simulink model "SAD_projectSamu"  (R2023b)
settings: Solver=ode4  StartTime=t0  StopTime=1000  FixedStep=t_step  RelTol=1e-3
model workspace (MAT data in the model file):
  N_order = 1
values from neighbouring files (symbols this model uses):
  A1 = importdata("igrfSg.txt")    [SAD_project_code.m]
  A2 = importdata("igrfSh.txt")    [SAD_project_code.m]
  A_1 = area_face(1)    [SAD_project_code.m]
  A_2 = area_face(2)    [SAD_project_code.m]
  A_3 = area_face(3)    [SAD_project_code.m]
  A_4 = area_face(4)    [SAD_project_code.m]
  A_5 = area_face(5)    [SAD_project_code.m]
  A_6 = area_face(6)    [SAD_project_code.m]
  alpha = [1/6 5/6]    [SAD_project_code.m]
  ARW = ARW*[1 1 1]'    [SAD_project_code.m]
  bias = bias*[1 1 1]'    [SAD_project_code.m]
  DCM_eci_per = rotationMatrix(rad2deg(i),rad2deg(OM), rad2deg(om))    [SAD_project_code.m]
  e = 0.0011241    [SAD_project_code.m]
  FS = 50000e-9    (= 5e-05)    [SAD_project_code.m]
  H0 = [g_10 g_11 h_11]'    [SAD_project_code.m]
  h_r_0 = [0,0,0]'    [SAD_project_code.m]
  horizon_cone_limit = deg2rad(350)    [SAD_project_code.m]
  I = 5/12.*diag([Ix Iy Iz])    [SAD_project_code.m]
  i = deg2rad(97.55)    [SAD_project_code.m]
  I_inv = inv(I)    [SAD_project_code.m]
  I_RW = 1e-2    (= 0.01)    [SAD_project_code.m]
  I_vector_RW = [I_RW I_RW I_RW]'    [SAD_project_code.m]
  inc_tot = sqrt(inc_lin^2 + inc_acc^2)    [SAD_project_code.m]
  InitialTrueAnomalyOfEarth = 0    [SAD_project_code.m]
  j_b = [0.001 0.005 0.001]'    [SAD_project_code.m]
  K1_point = lqr(A, B, Q, R)    [SAD_project_code.m]
  K1_slew = lqr(A,B, Q, R)    [SAD_project_code.m]
  K2_point = K1_point.^2/2    [SAD_project_code.m]
  K2_slew = K1_slew.^2/2    [SAD_project_code.m]
  K_detumbling = lqr(A,B,Q,R)    [SAD_project_code.m]
  matrix_RW_config = eye(3)    [SAD_project_code.m]
  matrix_RW_config_inv = inv(matrix_RW_config)    [SAD_project_code.m]
  mu_E = astroConstants(13)    [SAD_project_code.m]
  N_1 = BODY(1,:)    [SAD_project_code.m]
  N_2 = BODY(2,:)    [SAD_project_code.m]
  N_3 = BODY(3,:)    [SAD_project_code.m]
  N_4 = BODY(4,:)    [SAD_project_code.m]
  N_5 = BODY(5,:)    [SAD_project_code.m]
  N_6 = BODY(6,:)    [SAD_project_code.m]
  n_e = sqrt(mu_E/a^3)    [SAD_project_code.m]
  om = deg2rad(206.3209)    [SAD_project_code.m]
  OM = deg2rad(50.7464)    [SAD_project_code.m]
  p = a*(1-e^2)    [SAD_project_code.m]
  q0 = [0.1, -0.7, 0.51, 0.41]    [SAD_project_code.m]
  r_1 = r(1,:)    [SAD_project_code.m]
  r_2 = r(2,:)    [SAD_project_code.m]
  r_3 = r(3,:)    [SAD_project_code.m]
  r_4 = r(4,:)    [SAD_project_code.m]
  r_5 = r(5,:)    [SAD_project_code.m]
  r_6 = r(6,:)    [SAD_project_code.m]
  R_E = astroConstants(23)    [SAD_project_code.m]
  rho_d1 = 0.1    [SAD_project_code.m]
  rho_d2 = 0.1    [SAD_project_code.m]
  rho_d3 = 0.1    [SAD_project_code.m]
  rho_d4 = 0.1    [SAD_project_code.m]
  rho_d5 = 0.1    [SAD_project_code.m]
  rho_d6 = 0.1    [SAD_project_code.m]
  rho_s1 = rho_s(1)    [SAD_project_code.m]
  rho_s2 = rho_s(2)    [SAD_project_code.m]
  rho_s3 = rho_s(3)    [SAD_project_code.m]
  rho_s4 = rho_s(4)    [SAD_project_code.m]
  rho_s5 = rho_s(5)    [SAD_project_code.m]
  rho_s6 = rho_s(6)    [SAD_project_code.m]
  t_step = 0.01    [SAD_project_code.m]
  th0 = deg2rad(0)    [SAD_project_code.m]
  timeoflaunch = date2mjd2000(date0)    [SAD_project_code.m]
  torque_max = 0.8    [SAD_project_code.m]
  ts_sensor = 5*t_step    (= 0.05)    [SAD_project_code.m]
  w0 = [wx0 wy0 wz0]'    [SAD_project_code.m]
  w0_RW = [0 0 0]    [SAD_project_code.m]
  w_E = deg2rad(15.04)/60/60    [SAD_project_code.m]
  wMax_RW = 2*pi * RPM_max_RW / 60    (= 527.263967027)    [SAD_project_code.m]
libraries: matrix_library x43, dspindex x6, simulink x5, simulink_extras x4, sharedtransform x4, aerolibutil x2, vrlib x2, dspinverses x1
(part 4 of 4)

== system SAD_projectSamu/Attitude determination and sensoring/Subsystem1/Switch Case Action Only-Magnetometer/Subsystem/DCM to quaternion1 ==
  DCM : Inport
  Abs : Abs  SaturateOnIntegerOverflow=off
  Constant : Constant
  Demux : Demux
  Direction Cosine Matrix to Quaternions1 : sharedtransform/Direction Cosine Matrix  to Quaternions  aMode=0  action=None  tolerance=eps(2)
      settings: LibrarySourceBlock=|
      | aerolibtransform2/Direction Cosine Matrix
      | to Quaternions
  Divide : Product  Inputs=*/
  Extract Diagonal : matrix_library/Extract Diagonal
      settings: LibrarySourceBlock=|
      | simulink/Matrix
      | Operations/Extract Diagonal
  Gain : Gain  Gain=0.5
  Gain1 : Gain  Gain=[0 0 0; 0 0 1; 0 -1 0]
  Gain2 : Gain  Gain=[0 0 -1; 0 0 0; 1 0 0]
  Gain3 : Gain  Gain=[0 1 0; -1 0 0; 0 0 0]
  Gain4 : Gain  Gain=[4;4;4]
  MATLAB Function : MATLAB Function  TreatAsAtomicUnit=on
  Mux : Mux  Inputs=3
  Normalize Vector1 : Subsystem
  Sqrt : Sqrt
  Sum : Sum  Inputs=|++
  Sum of Elements{,1..3} (4 alike) : Sum  Inputs=+
  Unit Delay : UnitDelay  InitialCondition=q0  SampleTime=-1  HasFrameUpgradeWarning=on
  Vector Concatenate : Concatenate  NumInputs=3
  Vector Concatenate1 : Concatenate
  Vector Concatenate2 : Concatenate
  q (scalar last)1 : Outport
  wires:
  Extract Diagonal/1 -> Sum of Elements/1
  Sum of Elements/1 -> Sum/1
  Constant/1 -> Sum/2
  Sqrt/1 -> Gain/1
  ? -> Gain1/1, Gain2/1, Gain3/1, Extract Diagonal/1
  Gain2/1 -> Sum of Elements1/1
  Sum of Elements1/1 -> Vector Concatenate/2
  Gain1/1 -> Sum of Elements2/1
  Sum of Elements2/1 -> Vector Concatenate/1
  Sum of Elements3/1 -> Vector Concatenate/3
  Gain3/1 -> Sum of Elements3/1
  Vector Concatenate/1 -> Divide/1
  Gain/1 -> Vector Concatenate1/2, Gain4/1
  Divide/1 -> Vector Concatenate1/1
  Vector Concatenate1/1 -> Normalize Vector1/1(Vector)
  Sum/1 -> Abs/1
  Gain4/1 -> Divide/2
  Abs/1 -> Sqrt/1
  Direction Cosine Matrix to Quaternions1/1 -> Demux/1
  Demux/2 -> Mux/1
  Demux/3 -> Mux/2
  Demux/4 -> Mux/3
  Demux/1 -> Vector Concatenate2/2
  Mux/1 -> Vector Concatenate2/1
  DCM/1 -> Direction Cosine Matrix to Quaternions1/1
  Vector Concatenate2/1 -> MATLAB Function/1("quat ")
  Unit Delay/1 -> MATLAB Function/2(quat_last)
  MATLAB Function/1(quat) -> q (scalar last)1/1, Unit Delay/1

== system SAD_projectSamu/Attitude determination and sensoring/Subsystem1/Switch Case Action Only-Magnetometer/Subsystem/Norm vector ==
  Vector : Inport
  Dot Product : DotProduct  OutDataTypeStr=Inherit: Inherit via internal rule
  Sqrt : Sqrt
  Norm : Outport
  wires:
  Sqrt/1 -> Norm/1
  Vector/1 -> Dot Product/1, Dot Product/2
  Dot Product/1 -> Sqrt/1

== system SAD_projectSamu/Attitude determination and sensoring/Subsystem1/Switch Case Action Only-Magnetometer/Subsystem/Normalize Vector1 ==
  Vector : Inport
  Divide : Product  Inputs=*/
  Norm vector : Subsystem  AncestorBlock=LibrarySAD5/Normalize Vector1
  Versor : Outport
  wires:
  Vector/1 -> Norm vector/1(Vector), Divide/1
  Divide/1 -> Versor/1
  Norm vector/1(Norm) -> Divide/2

== system SAD_projectSamu/Attitude determination and sensoring/Subsystem1/Switch Case Action Only-Magnetometer/Subsystem/Normalize Vector5 ==
  Vector : Inport
  Divide : Product  Inputs=*/
  Norm vector : Subsystem  AncestorBlock=LibrarySAD5/Normalize Vector1
  Versor : Outport
  wires:
  Vector/1 -> Norm vector/1(Vector), Divide/1
  Divide/1 -> Versor/1
  Norm vector/1(Norm) -> Divide/2

== system SAD_projectSamu/Attitude determination and sensoring/Subsystem1/Switch Case Action Only-Magnetometer/Subsystem/Subsystem ==
  B_b versor : Inport
  Cross Product : matrix_library/Cross Product
  Cross Product1 : matrix_library/Cross Product
  Matrix Concatenate : Concatenate  NumInputs=3  Mode=Multidimensional array  ConcatenateDimension=2
  Matrix Multiply : Product  Multiplication=Matrix(*)
  Matrix Multiply1 : Product  Multiplication=Matrix(*)
  Normalize Vector1 : Subsystem
  Normalize Vector2 : Subsystem
  Normalize Vector6 : Subsystem
  Transpose : Math  Operator=transpose
  time derivative : Subsystem
  b_matrix : Outport
  wires:
  Matrix Multiply1/1 -> Normalize Vector1/1(Vector)  "b2 versor"
  B_b versor/1 -> Cross Product1/1, Matrix Concatenate/1, Matrix Multiply1/2, Cross Product/1, Matrix Multiply/1, time derivative/1(B_b versor)  "b1 versor"
  Transpose/1 -> Matrix Multiply/2
  Normalize Vector2/1(Versor) -> Matrix Concatenate/2, Cross Product1/2  "b3 versor"
  Matrix Multiply/1 -> Matrix Multiply1/1
  Cross Product/1 -> Normalize Vector2/1(Vector)
  Cross Product1/1 -> Normalize Vector6/1(Vector)
  Normalize Vector6/1(Versor) -> Matrix Concatenate/3  "b4 versor"
  Matrix Concatenate/1 -> b_matrix/1
  time derivative/1(B_b dot Versor) -> Transpose/1
  Normalize Vector1/1(Versor) -> Cross Product/2  "b3 versor"

== system SAD_projectSamu/Attitude determination and sensoring/Subsystem1/Switch Case Action Only-Magnetometer/Subsystem/Subsystem1 ==
  B_N versor : Inport
  Cross Product : matrix_library/Cross Product
  Cross Product1 : matrix_library/Cross Product
  Display : Display
  Display1 : Display
  Display2 : Display
  Matrix Concatenate : Concatenate  NumInputs=3  Mode=Multidimensional array  ConcatenateDimension=2
  Normalize Vector2 : Subsystem
  Normalize Vector6 : Subsystem
  time derivative : Subsystem
  r_matrix : Outport
  wires:
  time derivative/1(B_N dot Versor) -> Display/1, Cross Product/2  "r2 versor"
  B_N versor/1 -> Cross Product1/1, Matrix Concatenate/1, Display1/1, Cross Product/1, time derivative/1(B_N versor)  "r1 versor"
  Normalize Vector2/1(Versor) -> Matrix Concatenate/2, Cross Product1/2  "r3 versor"
  Cross Product/1 -> Display2/1, Normalize Vector2/1(Vector)
  Cross Product1/1 -> Normalize Vector6/1(Vector)
  Normalize Vector6/1(Versor) -> Matrix Concatenate/3  "r4 versor"
  Matrix Concatenate/1 -> r_matrix/1

== system SAD_projectSamu/Attitude determination and sensoring/Subsystem1/Switch Case Action Only-Magnetometer/Subsystem/time derivative ==
  B_b : Inport
  Gain1 : Gain  Gain=1/ ts_sensor
  Subtract : Sum  Inputs=+-
  Unit Delay : UnitDelay  InitialCondition=[0 0 0]'  SampleTime=-1  HasFrameUpgradeWarning=on
  B_b dot Versor : Outport
  wires:
  B_b/1 -> Subtract/1, Unit Delay/1
  Unit Delay/1 -> Subtract/2
  Subtract/1 -> Gain1/1  "B_b dot"
  Gain1/1 -> B_b dot Versor/1

== system SAD_projectSamu/Attitude determination and sensoring/Subsystem1/Switch Case Action Statisitcal Attitude/Create matrix to statistical method/Normalize Vector1 ==
  Vector : Inport
  Divide : Product  Inputs=*/
  Normalize Vector : Subsystem  AncestorBlock=LibrarySAD5/Normalize Vector1
  Versor : Outport
  wires:
  Vector/1 -> Normalize Vector/1(Vector), Divide/1
  Divide/1 -> Versor/1
  Normalize Vector/1(Norm) -> Divide/2

== system SAD_projectSamu/Attitude determination and sensoring/Subsystem1/Switch Case Action Statisitcal Attitude/Create matrix to statistical method/Normalize Vector2 ==
  Vector : Inport
  Divide : Product  Inputs=*/
  Normalize Vector : Subsystem  AncestorBlock=LibrarySAD5/Normalize Vector1
  Versor : Outport
  wires:
  Vector/1 -> Normalize Vector/1(Vector), Divide/1
  Divide/1 -> Versor/1
  Normalize Vector/1(Norm) -> Divide/2

== system SAD_projectSamu/Attitude determination and sensoring/Subsystem1/Switch Case Action Statisitcal Attitude/Create matrix to statistical method/Normalize Vector3 ==
  Vector : Inport
  Divide : Product  Inputs=*/
  Normalize Vector : Subsystem  AncestorBlock=LibrarySAD5/Normalize Vector1
  Versor : Outport
  wires:
  Vector/1 -> Normalize Vector/1(Vector), Divide/1
  Divide/1 -> Versor/1
  Normalize Vector/1(Norm) -> Divide/2

== system SAD_projectSamu/Attitude determination and sensoring/Subsystem1/Switch Case Action Statisitcal Attitude/Create matrix to statistical method/Normalize Vector4 ==
  Vector : Inport
  Divide : Product  Inputs=*/
  Normalize Vector : Subsystem  AncestorBlock=LibrarySAD5/Normalize Vector1
  Versor : Outport
  wires:
  Vector/1 -> Normalize Vector/1(Vector), Divide/1
  Divide/1 -> Versor/1
  Normalize Vector/1(Norm) -> Divide/2

== system SAD_projectSamu/Attitude determination and sensoring/Subsystem1/Switch Case Action Statisitcal Attitude/Statistical methods attitude determination (quaternion  Wabha’s problem) /For Iterator Subsystem to calculate B matrix ==
  note: Remember the last matrix B
  note: count the index
      | Important to flag reset in "State variable" to reset unit delay
  note: It's a for loop that resolve this expression
      | 𝐵 = ∑ 𝛼_𝑖*𝑠_𝑖*𝑣_𝑖' = [𝑏ij] to obatain matix B that it is a square matrix of order 3
      |
      | Analogous code for the iteration:
      |
      | for i = 1:size(alpha,2)
      | B = B + alpha(i)*s(:,i)*v(:,i)'
      | end
  alpha : Inport
  s matrix : Inport  Port=2
  v matrix : Inport  Port=3
  Add : Sum
  For Iterator : ForIterator  ResetStates=reset  IterationLimit=size(alpha,2)
  Matrix Multiply : Product  Multiplication=Matrix(*)
  Product : Product
  Transpose : Math  Operator=transpose
  Unit Delay1 : UnitDelay  SampleTime=-1  HasFrameUpgradeWarning=on
  Variable Selector : dspindex/Variable Selector  NumInputs=1  rowsOrCols=Columns  IdxMode=Variable  Elements=[1 3]  ZerOneIdxMode=One-based  errmode=Clip Index  FillMode=on  FillValues=0
  Variable Selector1 : dspindex/Variable Selector  NumInputs=1  rowsOrCols=Columns  IdxMode=Variable  Elements=[1 3]  ZerOneIdxMode=One-based  errmode=Clip Index  FillMode=on  FillValues=0
  Variable Selector2 : dspindex/Variable Selector  NumInputs=1  rowsOrCols=Columns  IdxMode=Variable  Elements=[1 3]  ZerOneIdxMode=One-based  errmode=Clip Index  FillMode=on  FillValues=0
  B matrix : Outport
  wires:
  For Iterator/1 -> Variable Selector1/2, Variable Selector/2, Variable Selector2/2
  alpha/1 -> Variable Selector2/1
  s matrix/1 -> Variable Selector/1
  Variable Selector2/1 -> Product/1
  Variable Selector/1 -> Product/2
  Product/1 -> Matrix Multiply/1
  Variable Selector1/1 -> Transpose/1
  Transpose/1 -> Matrix Multiply/2
  Matrix Multiply/1 -> Add/1
  v matrix/1 -> Variable Selector1/1
  Unit Delay1/1 -> Add/2
  Add/1 -> Unit Delay1/1, B matrix/1

== system SAD_projectSamu/Attitude determination and sensoring/Subsystem1/Switch Case Action Statisitcal Attitude/Statistical methods attitude determination (quaternion  Wabha’s problem) /Matrix trace ==
  Matrix : Inport
  Extract Diagonal : matrix_library/Extract Diagonal
      settings: LibrarySourceBlock=|
      | simulink/Matrix
      | Operations/Extract Diagonal
  Sum of Elements : Sum  Inputs=+
  trace : Outport
  wires:
  Extract Diagonal/1 -> Sum of Elements/1
  Sum of Elements/1 -> trace/1  "sigma"
  Matrix/1 -> Extract Diagonal/1

== system SAD_projectSamu/Attitude determination and sensoring/Subsystem1/Switch Case Action Statisitcal Attitude/Statistical methods attitude determination (quaternion  Wabha’s problem) /Vector z ==
  B : Inport
  Gain1 : Gain  Gain=-1
  Selector : Selector  NumberOfDimensions=2  InputPortWidth=3  IndexOptions=Index vector (dialog),Starting index (dialog)  Indices=2,3  OutputSizes=1,1
  Selector1 : Selector  NumberOfDimensions=2  InputPortWidth=3  IndexOptions=Index vector (dialog),Starting index (dialog)  Indices=1,3  OutputSizes=1,1
  Selector2 : Selector  NumberOfDimensions=2  InputPortWidth=3  IndexOptions=Index vector (dialog),Starting index (dialog)  Indices=1,2  OutputSizes=1,1
  Subtract1 : Sum  Inputs=+-
  Transpose1 : Math  Operator=transpose
  Vector Concatenate : Concatenate  NumInputs=3
  z : Outport
  wires:
  B/1 -> Subtract1/1, Transpose1/1
  Transpose1/1 -> Subtract1/2
  Selector2/1 -> Vector Concatenate/3
  Selector/1 -> Vector Concatenate/1
  Subtract1/1 -> Selector/1, Selector2/1, Selector1/1
  Vector Concatenate/1 -> z/1
  Gain1/1 -> Vector Concatenate/2
  Selector1/1 -> Gain1/1

== system SAD_projectSamu/Attitude determination and sensoring/Subsystem1/Switch Case Action Triad Case/DCM to quaternion1/Normalize Vector1 ==
  Vector : Inport
  Divide : Product  Inputs=*/
  Norm vector : Subsystem  AncestorBlock=LibrarySAD5/Normalize Vector1
  Versor : Outport
  wires:
  Vector/1 -> Norm vector/1(Vector), Divide/1
  Divide/1 -> Versor/1
  Norm vector/1(Norm) -> Divide/2

== system SAD_projectSamu/Attitude determination and sensoring/Subsystem1/Switch Case Action Triad Case/TRIAD: Attitude determination algebric Method with 2 sensor/Normalize Vector1 ==
  Vector : Inport
  Divide : Product  Inputs=*/
  Normalize Vector : Subsystem  AncestorBlock=LibrarySAD5/Normalize Vector1
  Versor : Outport
  wires:
  Vector/1 -> Normalize Vector/1(Vector), Divide/1
  Divide/1 -> Versor/1
  Normalize Vector/1(Norm) -> Divide/2

== system SAD_projectSamu/Attitude determination and sensoring/Subsystem1/Switch Case Action Triad Case/TRIAD: Attitude determination algebric Method with 2 sensor/Normalize Vector2 ==
  Vector : Inport
  Divide : Product  Inputs=*/
  Normalize Vector : Subsystem  AncestorBlock=LibrarySAD5/Normalize Vector1
  Versor : Outport
  wires:
  Vector/1 -> Normalize Vector/1(Vector), Divide/1
  Divide/1 -> Versor/1
  Normalize Vector/1(Norm) -> Divide/2

== system SAD_projectSamu/Attitude determination and sensoring/Subsystem1/Switch Case Action Triad Case/TRIAD: Attitude determination algebric Method with 2 sensor/Normalize Vector3 ==
  Vector : Inport
  Divide : Product  Inputs=*/
  Normalize Vector : Subsystem  AncestorBlock=LibrarySAD5/Normalize Vector1
  Versor : Outport
  wires:
  Vector/1 -> Normalize Vector/1(Vector), Divide/1
  Divide/1 -> Versor/1
  Normalize Vector/1(Norm) -> Divide/2

== system SAD_projectSamu/Attitude determination and sensoring/Subsystem1/Switch Case Action Triad Case/TRIAD: Attitude determination algebric Method with 2 sensor/Normalize Vector4 ==
  Vector : Inport
  Divide : Product  Inputs=*/
  Normalize Vector : Subsystem  AncestorBlock=LibrarySAD5/Normalize Vector1
  Versor : Outport
  wires:
  Vector/1 -> Normalize Vector/1(Vector), Divide/1
  Divide/1 -> Versor/1
  Normalize Vector/1(Norm) -> Divide/2

== system SAD_projectSamu/Attitude determination and sensoring/Subsystem1/Switch Case Action Triad Case/TRIAD: Attitude determination algebric Method with 2 sensor/Subsystem ==
  note: S1 = 𝑝;
      | 𝑠2 = (𝑝 ∧ 𝑞)/(|𝑝 ∧ 𝑞|);
      | 𝑠3 = 𝑝 ∧ 𝑠2
  versor p (body frame) : Inport
  versor q (body frame) : Inport  Port=2
  Cross Product : matrix_library/Cross Product
  Cross Product1 : matrix_library/Cross Product
  Matrix Concatenate : Concatenate  NumInputs=3  Mode=Multidimensional array  ConcatenateDimension=2
  Normalize Vector3 : Subsystem
  "Matrix S Measurements " : Outport
  wires:
  versor q (body frame)/1 -> Cross Product/2
  Normalize Vector3/1(Versor) -> Matrix Concatenate/2, Cross Product1/2  "s2"
  versor p (body frame)/1 -> Cross Product1/1, Matrix Concatenate/1, Cross Product/1  "s1"
  Cross Product/1 -> Normalize Vector3/1(Vector)
  Cross Product1/1 -> Matrix Concatenate/3  "s3"
  Matrix Concatenate/1 -> "Matrix S Measurements "/1  "Matrix of measure in body frame"

== system SAD_projectSamu/Attitude determination and sensoring/Subsystem1/Switch Case Action Triad Case/TRIAD: Attitude determination algebric Method with 2 sensor/Subsystem1 ==
  versor a (inertial) : Inport
  versor b (inertial) : Inport  Port=2
  Cross Product : matrix_library/Cross Product
  Cross Product1 : matrix_library/Cross Product
  Display : Display
  Matrix Concatenate : Concatenate  NumInputs=3  Mode=Multidimensional array  ConcatenateDimension=2
  Normalize Vector3 : Subsystem
  "Matrix V certain model " : Outport
  wires:
  versor b (inertial)/1 -> Cross Product/2
  Normalize Vector3/1(Versor) -> Matrix Concatenate/2, Cross Product1/2  "s2"
  versor a (inertial)/1 -> Cross Product1/1, Matrix Concatenate/1, Cross Product/1  "s1"
  Cross Product/1 -> Display/1, Normalize Vector3/1(Vector)
  Cross Product1/1 -> Matrix Concatenate/3  "s3"
  Matrix Concatenate/1 -> "Matrix V certain model "/1  "Matrix of measure in body frame"

== system SAD_projectSamu/Determine Control algorithm/Switch Case Action 3 axis stabilization Algorithm/DCM to quaternion1/Normalize Vector1/Norm vector ==
  Vector : Inport
  Dot Product : DotProduct  OutDataTypeStr=Inherit: Inherit via internal rule
  Sqrt : Sqrt
  Norm : Outport
  wires:
  Sqrt/1 -> Norm/1
  Vector/1 -> Dot Product/1, Dot Product/2
  Dot Product/1 -> Sqrt/1

== system SAD_projectSamu/Determine Control algorithm/Switch Case Action Slew Maneuver Algorithm/DCM to quaternion1/Normalize Vector1/Norm vector ==
  Vector : Inport
  Dot Product : DotProduct  OutDataTypeStr=Inherit: Inherit via internal rule
  Sqrt : Sqrt
  Norm : Outport
  wires:
  Sqrt/1 -> Norm/1
  Vector/1 -> Dot Product/1, Dot Product/2
  Dot Product/1 -> Sqrt/1

== system SAD_projectSamu/Enviroment Model/Magnetic Field/Switch Case Action Adavanced Magnetic model/Advanced magnetic field model/Rotation matrix for earth spin ==
  Clock1 : Clock
  Constant22 : Constant  Value=n_e
  Product3 : Product
  Rotation matrix 3 : Subsystem
  eci_to_ecef : Outport
  wires:
  Rotation matrix 3/1(theta_mat) -> eci_to_ecef/1
  Product3/1 -> Rotation matrix 3/1(In1)
  Constant22/1 -> Product3/1
  Clock1/1 -> Product3/2

== system SAD_projectSamu/Enviroment Model/Magnetic Field/Switch Case Action Adavanced Magnetic model/Advanced magnetic field model/cart to sph coord ==
  r_xyz : Inport
  Atan1 : Trigonometry  Operator=atan2
  Atan2 : Trigonometry  Operator=atan2
  Demux : Demux  Outputs=3
  Dot Product : DotProduct  OutDataTypeStr=Inherit: Inherit via internal rule
  Sqrt : Sqrt
  Square : Math  Operator=square
  Square Root : Sqrt
  Square1 : Math  Operator=square
  Sum : Sum  Inputs=|++
  r : Outport
  lat : Outport  Port=2
  long : Outport  Port=3
  wires:
  r_xyz/1 -> Dot Product/2, Dot Product/1, Demux/1
  Demux/2 -> Square/1, Atan2/1
  Demux/1 -> Atan2/2, Square1/1
  Atan2/1 -> long/1
  Demux/3 -> Atan1/1
  Square1/1 -> Sum/1
  Square/1 -> Sum/2
  Sum/1 -> Square Root/1
  Square Root/1 -> Atan1/2
  Atan1/1 -> lat/1
  Dot Product/1 -> Sqrt/1
  Sqrt/1 -> r/1

== system SAD_projectSamu/Enviroment Model/Magnetic Field/Switch Case Action Dipole model/Dipol Model of Magnetic Field/Calculation of b_n ==
  H0 vector : Inport
  EarthSat_n : Inport  Port=2
  Constant : Constant  Value=3
  Divide : Product  Inputs=*/
  Dot Product : DotProduct  OutDataTypeStr=Inherit: Inherit via internal rule
  Gain : Gain  Gain=3
  Gain1 : Gain  Gain=R_E^3
  Norm of Vector : Subsystem  AncestorBlock=LibrarySAD5/Normalize Vector1
  Norm of Vector H : Subsystem  AncestorBlock=LibrarySAD5/Normalize Vector1
  Normalize Vector : Subsystem
  Power : Math  Operator=pow
  Product : Product
  Product1 : Product
  Subtract : Sum  Inputs=+-
  m_versor : Subsystem
  b_N : Outport
  wires:
  Norm of Vector/1(Norm) -> Power/1
  Product/1 -> Subtract/1
  Divide/1 -> Gain1/1
  EarthSat_n/1 -> Norm of Vector/1(Vector), Normalize Vector/1(Vector)
  Normalize Vector/1(Versor) -> Product/1, Dot Product/1
  Gain1/1 -> Product1/1
  m_versor/1(m_versor) -> Dot Product/2, Subtract/2
  Gain/1 -> Product/2
  Product1/1 -> b_N/1
  Constant/1 -> Power/2
  Dot Product/1 -> Gain/1
  Subtract/1 -> Product1/2
  Norm of Vector H/1(Norm) -> Divide/1
  Power/1 -> Divide/2
  H0 vector/1 -> Norm of Vector H/1(Vector)

== system SAD_projectSamu/Subsystem/Subsystem/time derivative/Normalize Vector2/Norm vector ==
  Vector : Inport
  Dot Product : DotProduct  OutDataTypeStr=Inherit: Inherit via internal rule
  Sqrt : Sqrt
  Norm : Outport
  wires:
  Sqrt/1 -> Norm/1
  Vector/1 -> Dot Product/1, Dot Product/2
  Dot Product/1 -> Sqrt/1

== system SAD_projectSamu/Subsystem/Subsystem1/time derivative/Normalize Vector2/Norm vector ==
  Vector : Inport
  Dot Product : DotProduct  OutDataTypeStr=Inherit: Inherit via internal rule
  Sqrt : Sqrt
  Norm : Outport
  wires:
  Sqrt/1 -> Norm/1
  Vector/1 -> Dot Product/1, Dot Product/2
  Dot Product/1 -> Sqrt/1

== system SAD_projectSamu/Attitude determination and sensoring/Subsystem1/Switch Case Action Only-Magnetometer/Subsystem/DCM to quaternion1/Normalize Vector1 ==
  Vector : Inport
  Divide : Product  Inputs=*/
  Norm vector : Subsystem  AncestorBlock=LibrarySAD5/Normalize Vector1
  Versor : Outport
  wires:
  Vector/1 -> Norm vector/1(Vector), Divide/1
  Divide/1 -> Versor/1
  Norm vector/1(Norm) -> Divide/2

== system SAD_projectSamu/Attitude determination and sensoring/Subsystem1/Switch Case Action Only-Magnetometer/Subsystem/Normalize Vector1/Norm vector ==
  Vector : Inport
  Dot Product : DotProduct  OutDataTypeStr=Inherit: Inherit via internal rule
  Sqrt : Sqrt
  Norm : Outport
  wires:
  Sqrt/1 -> Norm/1
  Vector/1 -> Dot Product/1, Dot Product/2
  Dot Product/1 -> Sqrt/1

== system SAD_projectSamu/Attitude determination and sensoring/Subsystem1/Switch Case Action Only-Magnetometer/Subsystem/Normalize Vector5/Norm vector ==
  Vector : Inport
  Dot Product : DotProduct  OutDataTypeStr=Inherit: Inherit via internal rule
  Sqrt : Sqrt
  Norm : Outport
  wires:
  Sqrt/1 -> Norm/1
  Vector/1 -> Dot Product/1, Dot Product/2
  Dot Product/1 -> Sqrt/1

== system SAD_projectSamu/Attitude determination and sensoring/Subsystem1/Switch Case Action Only-Magnetometer/Subsystem/Subsystem/Normalize Vector1 ==
  Vector : Inport
  Display : Display
  Divide : Product  Inputs=*/
  Norm vector : Subsystem  AncestorBlock=LibrarySAD5/Normalize Vector1
  Versor : Outport
  wires:
  Vector/1 -> Norm vector/1(Vector), Divide/1
  Divide/1 -> Versor/1
  Norm vector/1(Norm) -> Display/1, Divide/2

== system SAD_projectSamu/Attitude determination and sensoring/Subsystem1/Switch Case Action Only-Magnetometer/Subsystem/Subsystem/Normalize Vector2 ==
  Vector : Inport
  Display : Display
  Divide : Product  Inputs=*/
  Norm vector : Subsystem  AncestorBlock=LibrarySAD5/Normalize Vector1
  Versor : Outport
  wires:
  Vector/1 -> Norm vector/1(Vector), Divide/1
  Divide/1 -> Versor/1
  Norm vector/1(Norm) -> Display/1, Divide/2

== system SAD_projectSamu/Attitude determination and sensoring/Subsystem1/Switch Case Action Only-Magnetometer/Subsystem/Subsystem/Normalize Vector6 ==
  Vector : Inport
  Divide : Product  Inputs=*/
  Norm vector : Subsystem  AncestorBlock=LibrarySAD5/Normalize Vector1
  Versor : Outport
  wires:
  Vector/1 -> Norm vector/1(Vector), Divide/1
  Divide/1 -> Versor/1
  Norm vector/1(Norm) -> Divide/2

== system SAD_projectSamu/Attitude determination and sensoring/Subsystem1/Switch Case Action Only-Magnetometer/Subsystem/Subsystem/time derivative ==
  B_b versor : Inport
  Gain1 : Gain  Gain=1/ ts_sensor
  Normalize Vector2 : Subsystem
  Subtract : Sum  Inputs=+-
  Unit Delay : UnitDelay  InitialCondition=[1 1 0]'  SampleTime=-1  HasFrameUpgradeWarning=on
  B_b dot Versor : Outport
  wires:
  B_b versor/1 -> Subtract/1, Unit Delay/1
  Unit Delay/1 -> Subtract/2
  Subtract/1 -> Gain1/1  "B_b dot"
  Normalize Vector2/1(Versor) -> B_b dot Versor/1
  Gain1/1 -> Normalize Vector2/1(Vector)

== system SAD_projectSamu/Attitude determination and sensoring/Subsystem1/Switch Case Action Only-Magnetometer/Subsystem/Subsystem1/Normalize Vector2 ==
  Vector : Inport
  Divide : Product  Inputs=*/
  Norm vector : Subsystem  AncestorBlock=LibrarySAD5/Normalize Vector1
  Versor : Outport
  wires:
  Vector/1 -> Norm vector/1(Vector), Divide/1
  Divide/1 -> Versor/1
  Norm vector/1(Norm) -> Divide/2

== system SAD_projectSamu/Attitude determination and sensoring/Subsystem1/Switch Case Action Only-Magnetometer/Subsystem/Subsystem1/Normalize Vector6 ==
  Vector : Inport
  Divide : Product  Inputs=*/
  Norm vector : Subsystem  AncestorBlock=LibrarySAD5/Normalize Vector1
  Versor : Outport
  wires:
  Vector/1 -> Norm vector/1(Vector), Divide/1
  Divide/1 -> Versor/1
  Norm vector/1(Norm) -> Divide/2

== system SAD_projectSamu/Attitude determination and sensoring/Subsystem1/Switch Case Action Only-Magnetometer/Subsystem/Subsystem1/time derivative ==
  B_N versor : Inport
  Gain1 : Gain  Gain=1/ ts_sensor
  Normalize Vector2 : Subsystem
  Subtract : Sum  Inputs=+-
  Unit Delay : UnitDelay  InitialCondition=[1 0 0]'  SampleTime=-1  HasFrameUpgradeWarning=on
  B_N dot Versor : Outport
  wires:
  B_N versor/1 -> Subtract/1, Unit Delay/1
  Unit Delay/1 -> Subtract/2
  Subtract/1 -> Gain1/1  "B_b dot"
  Normalize Vector2/1(Versor) -> B_N dot Versor/1
  Gain1/1 -> Normalize Vector2/1(Vector)

== system SAD_projectSamu/Attitude determination and sensoring/Subsystem1/Switch Case Action Statisitcal Attitude/Create matrix to statistical method/Normalize Vector1/Normalize Vector ==
  Vector : Inport
  Dot Product : DotProduct  OutDataTypeStr=Inherit: Inherit via internal rule
  Sqrt : Sqrt
  Norm : Outport
  wires:
  Sqrt/1 -> Norm/1
  Vector/1 -> Dot Product/1, Dot Product/2
  Dot Product/1 -> Sqrt/1

== system SAD_projectSamu/Attitude determination and sensoring/Subsystem1/Switch Case Action Statisitcal Attitude/Create matrix to statistical method/Normalize Vector2/Normalize Vector ==
  Vector : Inport
  Dot Product : DotProduct  OutDataTypeStr=Inherit: Inherit via internal rule
  Sqrt : Sqrt
  Norm : Outport
  wires:
  Sqrt/1 -> Norm/1
  Vector/1 -> Dot Product/1, Dot Product/2
  Dot Product/1 -> Sqrt/1

== system SAD_projectSamu/Attitude determination and sensoring/Subsystem1/Switch Case Action Statisitcal Attitude/Create matrix to statistical method/Normalize Vector3/Normalize Vector ==
  Vector : Inport
  Dot Product : DotProduct  OutDataTypeStr=Inherit: Inherit via internal rule
  Sqrt : Sqrt
  Norm : Outport
  wires:
  Sqrt/1 -> Norm/1
  Vector/1 -> Dot Product/1, Dot Product/2
  Dot Product/1 -> Sqrt/1

== system SAD_projectSamu/Attitude determination and sensoring/Subsystem1/Switch Case Action Statisitcal Attitude/Create matrix to statistical method/Normalize Vector4/Normalize Vector ==
  Vector : Inport
  Dot Product : DotProduct  OutDataTypeStr=Inherit: Inherit via internal rule
  Sqrt : Sqrt
  Norm : Outport
  wires:
  Sqrt/1 -> Norm/1
  Vector/1 -> Dot Product/1, Dot Product/2
  Dot Product/1 -> Sqrt/1

== system SAD_projectSamu/Attitude determination and sensoring/Subsystem1/Switch Case Action Triad Case/DCM to quaternion1/Normalize Vector1/Norm vector ==
  Vector : Inport
  Dot Product : DotProduct  OutDataTypeStr=Inherit: Inherit via internal rule
  Sqrt : Sqrt
  Norm : Outport
  wires:
  Sqrt/1 -> Norm/1
  Vector/1 -> Dot Product/1, Dot Product/2
  Dot Product/1 -> Sqrt/1

== system SAD_projectSamu/Attitude determination and sensoring/Subsystem1/Switch Case Action Triad Case/TRIAD: Attitude determination algebric Method with 2 sensor/Normalize Vector1/Normalize Vector ==
  Vector : Inport
  Dot Product : DotProduct  OutDataTypeStr=Inherit: Inherit via internal rule
  Sqrt : Sqrt
  Norm : Outport
  wires:
  Sqrt/1 -> Norm/1
  Vector/1 -> Dot Product/1, Dot Product/2
  Dot Product/1 -> Sqrt/1

== system SAD_projectSamu/Attitude determination and sensoring/Subsystem1/Switch Case Action Triad Case/TRIAD: Attitude determination algebric Method with 2 sensor/Normalize Vector2/Normalize Vector ==
  Vector : Inport
  Dot Product : DotProduct  OutDataTypeStr=Inherit: Inherit via internal rule
  Sqrt : Sqrt
  Norm : Outport
  wires:
  Sqrt/1 -> Norm/1
  Vector/1 -> Dot Product/1, Dot Product/2
  Dot Product/1 -> Sqrt/1

== system SAD_projectSamu/Attitude determination and sensoring/Subsystem1/Switch Case Action Triad Case/TRIAD: Attitude determination algebric Method with 2 sensor/Normalize Vector3/Normalize Vector ==
  Vector : Inport
  Dot Product : DotProduct  OutDataTypeStr=Inherit: Inherit via internal rule
  Sqrt : Sqrt
  Norm : Outport
  wires:
  Sqrt/1 -> Norm/1
  Vector/1 -> Dot Product/1, Dot Product/2
  Dot Product/1 -> Sqrt/1

== system SAD_projectSamu/Attitude determination and sensoring/Subsystem1/Switch Case Action Triad Case/TRIAD: Attitude determination algebric Method with 2 sensor/Normalize Vector4/Normalize Vector ==
  Vector : Inport
  Dot Product : DotProduct  OutDataTypeStr=Inherit: Inherit via internal rule
  Sqrt : Sqrt
  Norm : Outport
  wires:
  Sqrt/1 -> Norm/1
  Vector/1 -> Dot Product/1, Dot Product/2
  Dot Product/1 -> Sqrt/1

== system SAD_projectSamu/Attitude determination and sensoring/Subsystem1/Switch Case Action Triad Case/TRIAD: Attitude determination algebric Method with 2 sensor/Subsystem/Normalize Vector3 ==
  Vector : Inport
  Divide : Product  Inputs=*/
  Normalize Vector : Subsystem  AncestorBlock=LibrarySAD5/Normalize Vector1
  Versor : Outport
  wires:
  Vector/1 -> Normalize Vector/1(Vector), Divide/1
  Divide/1 -> Versor/1
  Normalize Vector/1(Norm) -> Divide/2

== system SAD_projectSamu/Attitude determination and sensoring/Subsystem1/Switch Case Action Triad Case/TRIAD: Attitude determination algebric Method with 2 sensor/Subsystem1/Normalize Vector3 ==
  Vector : Inport
  Divide : Product  Inputs=*/
  Normalize Vector : Subsystem  AncestorBlock=LibrarySAD5/Normalize Vector1
  Versor : Outport
  wires:
  Vector/1 -> Normalize Vector/1(Vector), Divide/1
  Divide/1 -> Versor/1
  Normalize Vector/1(Norm) -> Divide/2

== system SAD_projectSamu/Enviroment Model/Magnetic Field/Switch Case Action Adavanced Magnetic model/Advanced magnetic field model/Rotation matrix for earth spin/Rotation matrix 3 ==
  In1 : Inport
  Constant1 : Constant  Value=[0 0 0; 0 0 0; 0 0 1]
  Cos2 : Trigonometry  Operator=cos
  Gain : Gain  Gain=[1 0 0; 0 1 0; 0 0 0]
  Gain1 : Gain  Gain=[0 1 0; -1 0 0; 0 0 0]
  Sin2 : Trigonometry
  Sum : Sum  Inputs=+++
  theta_mat : Outport
  wires:
  Cos2/1 -> Gain/1
  Gain/1 -> Sum/1
  In1/1 -> Sin2/1, Cos2/1
  Sin2/1 -> Gain1/1
  Sum/1 -> theta_mat/1
  Gain1/1 -> Sum/2
  Constant1/1 -> Sum/3

== system SAD_projectSamu/Enviroment Model/Magnetic Field/Switch Case Action Dipole model/Dipol Model of Magnetic Field/Calculation of b_n/Norm of Vector ==
  Vector : Inport
  Dot Product : DotProduct  OutDataTypeStr=Inherit: Inherit via internal rule
  Sqrt : Sqrt
  Norm : Outport
  wires:
  Sqrt/1 -> Norm/1
  Vector/1 -> Dot Product/1, Dot Product/2
  Dot Product/1 -> Sqrt/1

== system SAD_projectSamu/Enviroment Model/Magnetic Field/Switch Case Action Dipole model/Dipol Model of Magnetic Field/Calculation of b_n/Norm of Vector H ==
  Vector : Inport
  Dot Product : DotProduct  OutDataTypeStr=Inherit: Inherit via internal rule
  Sqrt : Sqrt
  Norm : Outport
  wires:
  Sqrt/1 -> Norm/1
  Vector/1 -> Dot Product/1, Dot Product/2
  Dot Product/1 -> Sqrt/1

== system SAD_projectSamu/Enviroment Model/Magnetic Field/Switch Case Action Dipole model/Dipol Model of Magnetic Field/Calculation of b_n/Normalize Vector ==
  Vector : Inport
  Divide : Product  Inputs=*/
  Normalize Vector1 : Subsystem  AncestorBlock=LibrarySAD5/Normalize Vector1
  Versor : Outport
  wires:
  Vector/1 -> Normalize Vector1/1(Vector), Divide/1
  Divide/1 -> Versor/1
  Normalize Vector1/1(Norm) -> Divide/2

== system SAD_projectSamu/Enviroment Model/Magnetic Field/Switch Case Action Dipole model/Dipol Model of Magnetic Field/Calculation of b_n/m_versor ==
  Clock : Clock
  Constant : Constant  Value=cos(deg2rad(11.5))
  Cos : Trigonometry  Operator=cos
  Gain : Gain  Gain=deg2rad(w_E)
  Gain1 : Gain  Gain=sin(deg2rad(11.5))
  Gain2 : Gain  Gain=sin(deg2rad(11.5))
  Sin : Trigonometry
  Vector Concatenate : Concatenate  NumInputs=3
  m_versor : Outport
  wires:
  Clock/1 -> Gain/1
  Gain/1 -> Sin/1, Cos/1
  Gain2/1 -> Vector Concatenate/2
  Vector Concatenate/1 -> m_versor/1
  Cos/1 -> Gain1/1
  Constant/1 -> Vector Concatenate/3
  Sin/1 -> Gain2/1
  Gain1/1 -> Vector Concatenate/1

== system SAD_projectSamu/Attitude determination and sensoring/Subsystem1/Switch Case Action Only-Magnetometer/Subsystem/DCM to quaternion1/Normalize Vector1/Norm vector ==
  Vector : Inport
  Dot Product : DotProduct  OutDataTypeStr=Inherit: Inherit via internal rule
  Sqrt : Sqrt
  Norm : Outport
  wires:
  Sqrt/1 -> Norm/1
  Vector/1 -> Dot Product/1, Dot Product/2
  Dot Product/1 -> Sqrt/1

== system SAD_projectSamu/Attitude determination and sensoring/Subsystem1/Switch Case Action Only-Magnetometer/Subsystem/Subsystem/Normalize Vector1/Norm vector ==
  Vector : Inport
  Dot Product : DotProduct  OutDataTypeStr=Inherit: Inherit via internal rule
  Sqrt : Sqrt
  Norm : Outport
  wires:
  Sqrt/1 -> Norm/1
  Vector/1 -> Dot Product/1, Dot Product/2
  Dot Product/1 -> Sqrt/1

== system SAD_projectSamu/Attitude determination and sensoring/Subsystem1/Switch Case Action Only-Magnetometer/Subsystem/Subsystem/Normalize Vector2/Norm vector ==
  Vector : Inport
  Dot Product : DotProduct  OutDataTypeStr=Inherit: Inherit via internal rule
  Sqrt : Sqrt
  Norm : Outport
  wires:
  Sqrt/1 -> Norm/1
  Vector/1 -> Dot Product/1, Dot Product/2
  Dot Product/1 -> Sqrt/1

== system SAD_projectSamu/Attitude determination and sensoring/Subsystem1/Switch Case Action Only-Magnetometer/Subsystem/Subsystem/Normalize Vector6/Norm vector ==
  Vector : Inport
  Dot Product : DotProduct  OutDataTypeStr=Inherit: Inherit via internal rule
  Sqrt : Sqrt
  Norm : Outport
  wires:
  Sqrt/1 -> Norm/1
  Vector/1 -> Dot Product/1, Dot Product/2
  Dot Product/1 -> Sqrt/1

== system SAD_projectSamu/Attitude determination and sensoring/Subsystem1/Switch Case Action Only-Magnetometer/Subsystem/Subsystem/time derivative/Normalize Vector2 ==
  Vector : Inport
  Divide : Product  Inputs=*/
  Norm vector : Subsystem  AncestorBlock=LibrarySAD5/Normalize Vector1
  Versor : Outport
  wires:
  Vector/1 -> Norm vector/1(Vector), Divide/1
  Divide/1 -> Versor/1
  Norm vector/1(Norm) -> Divide/2

== system SAD_projectSamu/Attitude determination and sensoring/Subsystem1/Switch Case Action Only-Magnetometer/Subsystem/Subsystem1/Normalize Vector2/Norm vector ==
  Vector : Inport
  Dot Product : DotProduct  OutDataTypeStr=Inherit: Inherit via internal rule
  Sqrt : Sqrt
  Norm : Outport
  wires:
  Sqrt/1 -> Norm/1
  Vector/1 -> Dot Product/1, Dot Product/2
  Dot Product/1 -> Sqrt/1

== system SAD_projectSamu/Attitude determination and sensoring/Subsystem1/Switch Case Action Only-Magnetometer/Subsystem/Subsystem1/Normalize Vector6/Norm vector ==
  Vector : Inport
  Dot Product : DotProduct  OutDataTypeStr=Inherit: Inherit via internal rule
  Sqrt : Sqrt
  Norm : Outport
  wires:
  Sqrt/1 -> Norm/1
  Vector/1 -> Dot Product/1, Dot Product/2
  Dot Product/1 -> Sqrt/1

== system SAD_projectSamu/Attitude determination and sensoring/Subsystem1/Switch Case Action Only-Magnetometer/Subsystem/Subsystem1/time derivative/Normalize Vector2 ==
  Vector : Inport
  Divide : Product  Inputs=*/
  Norm vector : Subsystem  AncestorBlock=LibrarySAD5/Normalize Vector1
  Versor : Outport
  wires:
  Vector/1 -> Norm vector/1(Vector), Divide/1
  Divide/1 -> Versor/1
  Norm vector/1(Norm) -> Divide/2

== system SAD_projectSamu/Attitude determination and sensoring/Subsystem1/Switch Case Action Triad Case/TRIAD: Attitude determination algebric Method with 2 sensor/Subsystem/Normalize Vector3/Normalize Vector ==
  Vector : Inport
  Dot Product : DotProduct  OutDataTypeStr=Inherit: Inherit via internal rule
  Sqrt : Sqrt
  Norm : Outport
  wires:
  Sqrt/1 -> Norm/1
  Vector/1 -> Dot Product/1, Dot Product/2
  Dot Product/1 -> Sqrt/1

== system SAD_projectSamu/Attitude determination and sensoring/Subsystem1/Switch Case Action Triad Case/TRIAD: Attitude determination algebric Method with 2 sensor/Subsystem1/Normalize Vector3/Normalize Vector ==
  Vector : Inport
  Dot Product : DotProduct  OutDataTypeStr=Inherit: Inherit via internal rule
  Sqrt : Sqrt
  Norm : Outport
  wires:
  Sqrt/1 -> Norm/1
  Vector/1 -> Dot Product/1, Dot Product/2
  Dot Product/1 -> Sqrt/1

== system SAD_projectSamu/Enviroment Model/Magnetic Field/Switch Case Action Dipole model/Dipol Model of Magnetic Field/Calculation of b_n/Normalize Vector/Normalize Vector1 ==
  Vector : Inport
  Dot Product : DotProduct  OutDataTypeStr=Inherit: Inherit via internal rule
  Sqrt : Sqrt
  Norm : Outport
  wires:
  Sqrt/1 -> Norm/1
  Vector/1 -> Dot Product/1, Dot Product/2
  Dot Product/1 -> Sqrt/1

== system SAD_projectSamu/Attitude determination and sensoring/Subsystem1/Switch Case Action Only-Magnetometer/Subsystem/Subsystem/time derivative/Normalize Vector2/Norm vector ==
  Vector : Inport
  Dot Product : DotProduct  OutDataTypeStr=Inherit: Inherit via internal rule
  Sqrt : Sqrt
  Norm : Outport
  wires:
  Sqrt/1 -> Norm/1
  Vector/1 -> Dot Product/1, Dot Product/2
  Dot Product/1 -> Sqrt/1

== system SAD_projectSamu/Attitude determination and sensoring/Subsystem1/Switch Case Action Only-Magnetometer/Subsystem/Subsystem1/time derivative/Normalize Vector2/Norm vector ==
  Vector : Inport
  Dot Product : DotProduct  OutDataTypeStr=Inherit: Inherit via internal rule
  Sqrt : Sqrt
  Norm : Outport
  wires:
  Sqrt/1 -> Norm/1
  Vector/1 -> Dot Product/1, Dot Product/2
  Dot Product/1 -> Sqrt/1

== matlab function SAD_projectSamu/Enviroment Model/Magnetic Field/Switch Case Action Adavanced Magnetic model/Advanced magnetic field model/MATLAB Function ==
  data: r input; B_n output; theta input; phi input; LST input; mjd2000 input; A1 input; A2 input; N input
function B_n = magnetic_field_model(r,theta,phi, LST, mjd2000, A1, A2, N)

%   mjd2000[1]  Date in MJD 2000. MJD2000 is defined as the number of days
%               since 01-01-2000, 12:00 noon.
days = mjd2000 - 7305;      % 7305 is the Julian time from 2000 to 2020

% Inputs
% r         Geocentric radius
% theta     Latitude measured in degrees positive from equator  
% phi       Longitude measured in degrees positive east from Greenwich
% days      Decimal days since January 1, 2020
% N         Order of expansion of the magnetic field model
%
% Outputs - magnetic field strength in local tangential coordinates
% Br    B in radial direction
% Bt    B in theta direction
% Bp    B in phi direction
[Br,Bt,Bp] = magnet(r,theta,phi,days, N, A1, A2);

% Inputs
% Br    B in radial direction
% Bt    B in theta direction
% Bp    B in phi direction
% LST   Local sidereal time of location (in degrees)(right ascension)
% lat   Latitude measured positive north from equator (in degrees), it is
%       the same as the local declination
%
% Outputs
% Bx    B in x-direction  | Magnetic field strength (B)
% By    B in y-direction  | in geocentric inertial coordinates
% Bz    B in z-direction  |
[Bx,By,Bz] = msph2inert(Br,Bt,Bp,LST, theta);

B_n = [Bx,By,Bz]';

== matlab function SAD_projectSamu/Statistical methods attitude determination (quaternion  Wabha’s problem) /Blocco da convertire in formato simulink. Ho trovato 3 soluzioni differenti al proble ==
  data: K input; q output; S input; Sadj input
function q = fcn(K, S, Sadj)
    
    A = eig(K);
    A = real(A);
    lambda = max(A);
    z = K(1:3, 4);

    %{
    FUNZIONAAA
    %proposta wikipedia
    sigma = 1/2*trace(S);
    %Sadj = det(S)*eye(3)*inv(S);
    k = trace(Sadj);
    delta = det(S);
    alpha = lambda^2 - sigma^2 + k;
    beta = lambda - sigma;
    gamma = (lambda + sigma)*alpha - delta;
    
    x = (alpha*eye(3) + beta*S + S^2)*z;
    
    q =[x; gamma]/sqrt(gamma^2 + norm(x)^2);
    %}
   
    %
    %Proposta libro: FUNZIONAAAAAA -> sceglierei questa: è facile da
    %implementare
    
    z = K(1:3, 4);
    sigma = K(4,4);
    
    mat = (lambda + sigma)*eye(3) - S;
    q = zeros(4,1);
    q(1:3) = (det(mat)*eye(3)*inv(mat)) * z;
    q(4) = det(mat);
    q = q/norm(q);
    %}


    %{
    GIUSTA FUNZIONA, ma restituisce gibbs vector
    z = K(1:3, 4);
    sigma = K(4,4);
    %K = K - eye(4)*lambda;
    
    % linear system
    %Z = zeros(4,1);
    %q = K\Z;
    %q = q/norm(q);
    
    g = (S-(sigma+lambda)*eye(3)) \ (-z);
    
    DCM = [1+g(1)^2-g(2)^2-g(3)^2, 2*(g(1)*g(2)+g(3))    ,  2*(g(1)*g(3)-g(2));
         2*(g(1)*g(2)-g(3))    , 1-g(1)^2+g(2)^2-g(3)^2,  2*(g(2)*g(3)+g(1));
         2*(g(1)*g(3)+g(2))    , 2*(g(2)*g(3)-g(1))    ,  1-g(1)^2-g(2)^2+g(3)^2];
    DCM = DCM./(1+g(1)^2+g(2)^2+g(3)^2);
    %}

    %{
    % soluzione nelle slide, ma la matrice è singolare
    q = (K - lambda*eye(4)) \ zeros(4,1);
    q = q/norm(q);
    %}

end

== matlab function SAD_projectSamu/Attitude determination and sensoring/Subsystem1/Switch Case Action Statisitcal Attitude/Statistical methods attitude determination (quaternion  Wabha’s problem) /Blocco da convertire in formato simulink. Ho trovato 3 soluzioni differenti al proble ==
  data: K input; q output; S input; Sadj input
function q = fcn(K, S, Sadj)
    
    A = eig(K);
    A = real(A);
    lambda = max(A);
    z = K(1:3, 4);

    %{
    FUNZIONAAA
    %proposta wikipedia
    sigma = 1/2*trace(S);
    %Sadj = det(S)*eye(3)*inv(S);
    k = trace(Sadj);
    delta = det(S);
    alpha = lambda^2 - sigma^2 + k;
    beta = lambda - sigma;
    gamma = (lambda + sigma)*alpha - delta;
    
    x = (alpha*eye(3) + beta*S + S^2)*z;
    
    q =[x; gamma]/sqrt(gamma^2 + norm(x)^2);
    %}
   
    %
    %Proposta libro: FUNZIONAAAAAA -> sceglierei questa: è facile da
    %implementare
    
    z = K(1:3, 4);
    sigma = K(4,4);
    
    mat = (lambda + sigma)*eye(3) - S;
    q = zeros(4,1);
    q(1:3) = (det(mat)*eye(3)*inv(mat)) * z;
    q(4) = det(mat);
    q = q/norm(q);
    %}


    %{
    GIUSTA FUNZIONA, ma restituisce gibbs vector
    z = K(1:3, 4);
    sigma = K(4,4);
    %K = K - eye(4)*lambda;
    
    % linear system
    %Z = zeros(4,1);
    %q = K\Z;
    %q = q/norm(q);
    
    g = (S-(sigma+lambda)*eye(3)) \ (-z);
    
    DCM = [1+g(1)^2-g(2)^2-g(3)^2, 2*(g(1)*g(2)+g(3))    ,  2*(g(1)*g(3)-g(2));
         2*(g(1)*g(2)-g(3))    , 1-g(1)^2+g(2)^2-g(3)^2,  2*(g(2)*g(3)+g(1));
         2*(g(1)*g(3)+g(2))    , 2*(g(2)*g(3)-g(1))    ,  1-g(1)^2-g(2)^2+g(3)^2];
    DCM = DCM./(1+g(1)^2+g(2)^2+g(3)^2);
    %}

    %{
    % soluzione nelle slide, ma la matrice è singolare
    q = (K - lambda*eye(4)) \ zeros(4,1);
    q = q/norm(q);
    %}

end

== matlab function SAD_projectSamu/Determine Control algorithm/Switch Case Action 3 axis stabilization Algorithm/DCM to quaternion1/MATLAB Function ==
  data: quat input; quat output; quat_last input
function quat = fcn(quat, quat_last)

[~,x] = max(abs(quat_last));  % Pick off index of max abs of last quaternion
if( quat(x)*quat_last(x) < 0 )  % If sign changed ...
    quat = -quat;  % Flip all signs
end

== matlab function SAD_projectSamu/Attitude determination and sensoring/Subsystem1/Switch Case Action Only-Magnetometer/Subsystem/DCM to quaternion1/MATLAB Function ==
  data: quat input; quat output; quat_last input
function quat = fcn(quat, quat_last)

[~,x] = max(abs(quat_last));  % Pick off index of max abs of last quaternion
if( quat(x)*quat_last(x) < 0 )  % If sign changed ...
    quat = -quat;  % Flip all signs
end

== matlab function SAD_projectSamu/Attitude determination and sensoring/Subsystem1/Switch Case Action Triad Case/DCM to quaternion1/MATLAB Function ==
  data: quat input; quat output; quat_last input
function quat = fcn(quat, quat_last)

[~,x] = max(abs(quat_last));  % Pick off index of max abs of last quaternion
if( quat(x)*quat_last(x) < 0 )  % If sign changed ...
    quat = -quat;  % Flip all signs
end

== matlab function SAD_projectSamu/Determine Control algorithm/Switch Case Action Slew Maneuver Algorithm/DCM to quaternion1/MATLAB Function ==
  data: quat input; quat output; quat_last input
function quat = fcn(quat, quat_last)

[~,x] = max(abs(quat_last));  % Pick off index of max abs of last quaternion
if( quat(x)*quat_last(x) < 0 )  % If sign changed ...
    quat = -quat;  % Flip all signs
end
